simulink model "qbot2_sim_2019b"  (R2019b)
settings: Solver=FixedStepAuto  StartTime=0.0  StopTime=P.t_end  FixedStep=P.dt  RelTol=1e-3
InitFcn:
  | % load_qbot2_sim
StopFcn:
  | if (P.plotsim_flag)
  |     plot_sim(out, P)
  | end
(part 2 of 2)

== matlab function qbot2_sim_2019b/PVA Error State Estimation/Kalman Filter ==
  data: t_k input; f_b__i_b input; C_t__b input; v_t__t_b input; delta_r_t__t_b output; delta_v_t__t_b output; delta_C_t__b output; z_k_1 input; z_k_2 input; sigma_SNHT input; z_k_3 input; P parameter; P_posteriori_k output; residuals output; K output
function [delta_r_t__t_b, delta_v_t__t_b, delta_C_t__b, P_posteriori_k, residuals, K] = ...
              IMU_Error_State_Estimation(t_k, f_b__i_b, C_t__b, v_t__t_b, z_k_1, z_k_2, sigma_SNHT, z_k_3, P)

%% IMU Error State Estimation Function
% Recieves error measurements from the difference between odometry and the
% IMU, and provides estimates of that error.  

% Build randn quantities from etrinsic functions
coder.extrinsic('randn');

persistent x_posteriori_k_1 P_posteriori_k_1 A Q_bar K_prev

dt = P.dt;

% Normalize C_t__b_est
C_t__b = q2dcm(dcm2q(C_t__b));

%**************************************************************************
%% Kalman Filter Prediction Steps
%**************************************************************************

% For first instance only
if (isempty(x_posteriori_k_1))
    
    % Build Random Vector
    rand_vec = zeros(6,1);
    rand_vec = randn(6,1);
    
    % Set Initial Values for x and P_______________________________________
    P_0 = diag([5 * pi/180; 5 * pi/180; 5 * pi/180; ... % Initial Attitude Uncertianty (Angle-Axis)
                0.5; 0.5; 0.5; ...                      % Initial Velocity Uncertianty
                1.5; 1.5; 1.5; ...                      % Initial Position Uncertianty 
                10 * P.accel.BI.sigma_n; ...            % Initial Accel Bias Instability Uncertianty
                10 * P.gyro.BI.sigma_n] .^ 2);          % Initial Gyro Bias Instability Uncertianty
    x_0 = [z_k_2; ...                      % First measurement of attitude error
           z_k_1;   ...                    % First measurement of velocity error
           0; 0; 0;    ...                 % {t} frame always starts at zero
           ((P_0(10:15,10:15) / 10) * rand_vec)]; % Bias Instabilities drawn from distribution
    x_posteriori_k_1 = zeros(15,1);
    P_posteriori_k_1 = eye(15);
    
    K_prev = zeros(15,3);
    
    % Build the Contiuous Time Model_______________________________________
    A = zeros(15, 15);
    
    % Compute A - Fifth Row
    A(13:15, 13:15) = -eye(3) ./ P.gyro.BI.correlation_time;
    
    % Compute A - Fourth Row
    A(10:12, 10:12) = -eye(3) ./ P.accel.BI.correlation_time;
    
    % Compute A - Third Row
    A(7:9, 4:6) = eye(3);
    
    % Compute A - Second Row
    A(4:6, 1:3) = -vec2ss(C_t__b * f_b__i_b);
    A(4:6, 4:6) = -2 .* P.Ohm_t__i_e;
    A(4:6, 10:12) = -C_t__b;

    % Compute the monstrosity A(4:6, 7:9) a.k.a. A_23
    r_e__e_b_hat = P.r_e__e_t; % initial position is always the origin
    [L_b_hat, ~, ~] = xyz2llh(r_e__e_b_hat, P);
    g_0 = Somigliana(L_b_hat, P);
    r_e__e_S = Geo_Radius(L_b_hat, P);
    A(4:6, 7:9) = P.C_e__t' * ((2 * g_0 * r_e__e_b_hat) / ...
                 (r_e__e_S * norm(r_e__e_b_hat)^2)) * ...
                  r_e__e_b_hat' * P.C_e__t;
    
    % Compute A - First Row
    A(1:3, 1:3) = -P.Ohm_t__i_e;
    A(1:3, 13:15) = -C_t__b;
    
    % Define Q_bar_________________________________________________________
    Q_vec = [P.gyro.sigma_ARW.^2;   ...       % Attitude Process Noise rad/s
             P.accel.sigma_VRW.^2;  ...       % Velocity Process Noise m/s
             zeros(3,1);         ...          % Position Process Noise
             P.accel.BI.sigma_n.^2; ...       % Accel Bias Instability Process Noise m/s
             P.gyro.BI.sigma_n.^2];           % Gyro  Bias Instability Process Noise rad/s
     
    % Allow for a margin of error for tuning     
    Q_fudge_factor = 1;
    
    % Set Q
    Q_bar = diag(Q_fudge_factor .* Q_vec');
    
    % Discritize the Continuous Time Model_________________________________
    F = eye(15) + A*dt;
    Q = (1/2) * ((F*Q_bar*F') + Q_bar) * dt;
    
    % Compute first prediction_____________________________________________
    x_priori_k = F * x_0;
    P_priori_k = (F * P_0 * F') + Q;
    
%__________________________________________________________________________
% All other instances: State Prediction  
else
    
    % Re-compute the time varying arguements of A__________________________

    % Compute A - Second Row
    A(4:6, 1:3) = -vec2ss(C_t__b * f_b__i_b);
    A(4:6, 10:12) = -C_t__b;
    
    % Compute A - First Row
    A(1:3, 13:15) = -C_t__b;
    
    % Discritize the Continuous Time Model_________________________________
    F = eye(15) + A*dt;
    Q = (1/2) * ((F*Q_bar*F') + Q_bar) * dt;
    
    % Compute prediction step
    x_priori_k = (F * x_posteriori_k_1);
    P_priori_k = (F * P_posteriori_k_1 * F') + Q;
    
    % Symmetrisize P
    P_priori_k = (P_priori_k + P_priori_k') / 2;
    
end

%**************************************************************************
%% Kalman Filter Measurement Update Steps
%**************************************************************************
% This section is segmented according to the aiding sensor configuration

%__________________________________________________________________________
% No Measurement Updates
if (P.aiding_sensor_config == 0)
    
    x_posteriori_k = x_priori_k;
    P_posteriori_k = P_priori_k;
    residuals = zeros(3,1);
    K = zeros(15,3);
    
%__________________________________________________________________________
% Fake Velocity Aiding Only
elseif (P.aiding_sensor_config == 1)
    
    % Set H Matrix -- H = [(v_t__t_b,x), I_3, 0_3, 0_3, 0_3]
    H = [vec2ss(v_t__t_b), eye(3), zeros(3,9)]; 
    
    % Define R with known sigmas
    R_vec = P.sigma_fake_v .^ 2;
    R = diag(R_vec);
    
    % Kalman Gain Computation
    K = (P_priori_k * H') / (H * P_priori_k * H' + R);
    
    % Compute Residuals
    residuals = z_k_1 - H*x_priori_k;
    
    % A Posteriori State and Covariance Update
    x_posteriori_k = x_priori_k + K*(z_k_1 - H*x_priori_k);
    P_posteriori_k = (eye(15) - K*H) * P_priori_k;
    
    %Symmetrisize P
    P_posteriori_k = (P_posteriori_k + P_posteriori_k') / 2;
    

%__________________________________________________________________________
% Fake Attitude Only
elseif (P.aiding_sensor_config == 2)
    
    % Only Update at a frequency of 1 Hz
    if (mod(t_k, 1) == 0)
        
        % Set H Matrix -- H = [I_3, 0_3, 0_3, 0_3, 0_3]
        H = [eye(3), zeros(3,12)];
        
        % Define R with known sigmas
        R_vec = P.sigma_fake_psi .^ 2;
        R = diag(R_vec);
        
        % Kalman Gain Computation
        K = (P_priori_k * H') / (H * P_priori_k * H' + R);
        
        % Compute Residuals
        residuals = z_k_2 - H*x_priori_k;
        
        % A Posteriori State and Covariance Update
        x_posteriori_k = x_priori_k + K*(z_k_2 - H*x_priori_k);
        P_posteriori_k = (eye(15) - K*H) * P_priori_k;
        
        %Symmetrisize P
        P_posteriori_k = (P_posteriori_k + P_posteriori_k') / 2;
        
        % Save Value of K_prev
        K_prev = K;
    
    % No measurement update at this time step
    else
        
        % Carry Through
        x_posteriori_k = x_priori_k;
        P_posteriori_k = P_priori_k;
        residuals = zeros(3,1);
        K = K_prev;
       
    end
    

%__________________________________________________________________________
% Full Fake Attitude (Velocity & Attitude)
elseif (P.aiding_sensor_config == 3)
    
    % Velocity Update at every time step
    
    % Set H Matrix -- H = [(v_t__t_b,x), I_3, 0_3, 0_3, 0_3]
    H = [vec2ss(v_t__t_b), eye(3), zeros(3,9)];
    
    % Define R with known sigmas
    R_vec = P.sigma_fake_v .^ 2;
    R = diag(R_vec);
    
    % Kalman Gain Computation
    K = (P_priori_k * H') / (H * P_priori_k * H' + R);
    
    % Compute Residuals
    residuals = z_k_1 - H*x_priori_k;
    
    % A Posteriori State and Covariance Update
    x_posteriori_k = x_priori_k + K*(z_k_1 - H*x_priori_k);
    P_posteriori_k = (eye(15) - K*H) * P_priori_k;
    
    %Symmetrisize P
    P_posteriori_k = (P_posteriori_k + P_posteriori_k') / 2;
    
    %- - - - - - - - - - - - - - - - - - - - - - - - - - - - - - - - - - -
    % Attitude Update at a frequency of 1 Hz
    if (mod(t_k, 1) == 0)
        
        % Set H Matrix -- H = [I_3, 0_3, 0_3, 0_3, 0_3]
        H = [eye(3), zeros(3,12)];
        
        % Define R with known sigmas
        R_vec = P.sigma_fake_psi .^ 2;
        R = diag(R_vec);
        
        % Kalman Gain Computation
        K = (P_priori_k * H') / (H * P_priori_k * H' + R);
        
        % Compute Residuals
        residuals = z_k_2 - H*x_priori_k;
        
        % A Posteriori State and Covariance Update
        x_posteriori_k = x_priori_k + K*(z_k_2 - H*x_priori_k);
        P_posteriori_k = (eye(15) - K*H) * P_priori_k;
        
        %Symmetrisize P
        P_posteriori_k = (P_posteriori_k + P_posteriori_k') / 2;
        
        % Save Value of K_prev
        K_prev = K;
        
    end
    %- - - - - - - - - - - - - - - - - - - - - - - - - - - - - - - - - - -
    
%__________________________________________________________________________
% Odometry Aiding Only
elseif (P.aiding_sensor_config == 4)
    
    % Set H Matrix -- H = [(v_t__t_b,x), I_3, 0_3, 0_3, 0_3]
    H = [vec2ss(v_t__t_b), eye(3), zeros(3,9)]; 
    
    % Define R Vector
    R_b_vec = P.sigma_v_b__t_b_odo .^ 2;
    
    % Build the R Matrix
    R = C_t__b * diag(R_b_vec) * C_t__b';
    
    % Kalman Gain Computation
    K = (P_priori_k * H') / (H * P_priori_k * H' + R);
    
    % Compute Residuals
    residuals = z_k_1 - H*x_priori_k;
    
    % A Posteriori State and Covariance Update
    x_posteriori_k = x_priori_k + K*(z_k_1 - H*x_priori_k);
    P_posteriori_k = (eye(15) - K*H) * P_priori_k;
    
    %Symmetrisize P
    P_posteriori_k = (P_posteriori_k + P_posteriori_k') / 2;
    
%__________________________________________________________________________
% Kinect Camera Attitude Only
elseif (P.aiding_sensor_config == 5)
    
    % Only Update at a frequency of 1 Hz
    if (mod(t_k, 1) == 0)
        
        % Set H Matrix -- H = [I_3, 0_3, 0_3, 0_3, 0_3]
        H = [eye(3), zeros(3,12)];
        
        % Compute Jacobian
        [~, pitch, roll] = dcm2ypr(C_t__b);
        J = [1, 0, -sin(pitch); ...
             0, cos(roll), sin(roll)*cos(pitch); ...
             0, -sin(roll), cos(roll)*cos(pitch)];
        
        % Define R_e with known sigmas
        R_e = diag(sigma_SNHT .^ 2);
        
        % Convert R_e to R_k
        R_k = J * R_e * J';
        
        % Kalman Gain Computation
        K = (P_priori_k * H') / (H * P_priori_k * H' + R_k);
        
        % Compute Residuals
        residuals = z_k_2 - H*x_priori_k;
        
        % A Posteriori State and Covariance Update
        x_posteriori_k = x_priori_k + K*(z_k_2 - H*x_priori_k);
        P_posteriori_k = (eye(15) - K*H) * P_priori_k;
        
        %Symmetrisize P
        P_posteriori_k = (P_posteriori_k + P_posteriori_k') / 2;
        
        % Save Value of K_prev
        K_prev = K;
    
    % No measurement update at this time step
    else
        
        % Carry Through
        x_posteriori_k = x_priori_k;
        P_posteriori_k = P_priori_k;
        residuals = zeros(3,1);
        K = K_prev;
       
    end    

%__________________________________________________________________________
% Full Aiding (Odometry & Kinect Camera)
elseif (P.aiding_sensor_config == 6)
    
    % Velocity Update at every time step
    
    % Set H Matrix -- H = [(v_t__t_b,x), I_3, 0_3, 0_3, 0_3]
    H = [vec2ss(v_t__t_b), eye(3), zeros(3,9)];
    
    % Compute Jacobian
    [~, pitch, roll] = dcm2ypr(C_t__b);
    J = [1, 0, -sin(pitch); ...
         0, cos(roll), sin(roll)*cos(pitch); ...
         0, -sin(roll), cos(roll)*cos(pitch)];
    
    % Define R_e with known sigmas
    R_e = diag(sigma_SNHT .^ 2);
    
    % Convert R_e to R_k
    R_k = J * R_e * J';
    
    % Kalman Gain Computation
    K = (P_priori_k * H') / (H * P_priori_k * H' + R_k);
    
    % Compute Residuals
    residuals = z_k_1 - H*x_priori_k;
    
    % A Posteriori State and Covariance Update
    x_posteriori_k = x_priori_k + K*(z_k_1 - H*x_priori_k);
    P_posteriori_k = (eye(15) - K*H) * P_priori_k;
    
    %Symmetrisize P
    P_posteriori_k = (P_posteriori_k + P_posteriori_k') / 2;
    
    %- - - - - - - - - - - - - - - - - - - - - - - - - - - - - - - - - - -
    % Attitude Update at a frequency of 1 Hz
    if (mod(t_k, 1) == 0)
        
        % Set H Matrix -- H = [I_3, 0_3, 0_3, 0_3, 0_3]
        H = [eye(3), zeros(3,12)];
        
        % Define R with known sigmas
        R_vec = P.sigma_SNHT .^ 2;
        R = diag(R_vec);
        
        % Kalman Gain Computation
        K = (P_priori_k * H') / (H * P_priori_k * H' + R);
        
        % Compute Residuals
        residuals = z_k_2 - H*x_priori_k;
        
        % A Posteriori State and Covariance Update
        x_posteriori_k = x_priori_k + K*(z_k_2 - H*x_priori_k);
        P_posteriori_k = (eye(15) - K*H) * P_priori_k;
        
        %Symmetrisize P
        P_posteriori_k = (P_posteriori_k + P_posteriori_k') / 2;
        
        % Save Value of K_prev
        K_prev = K;
        
    end
    %- - - - - - - - - - - - - - - - - - - - - - - - - - - - - - - - - - -    
    
end

%__________________________________________________________________________
%% Barometer as an Aiding Sensor

if (P.use_barometer == true)
    
    % Set H (this is done as a one-dimensional case)
    H = 1;
    
    % Build the R Matrix
    R = P.sigma_baro^2 * 1.3;
    
    % Kalman Gain Computation
    P_priori_z = P_posteriori_k(9,9);
    K_baro = (P_priori_z * H') / (H * P_priori_z * H' + R);
    
    % A Posteriori State and Covariance Update
    x_posteriori_k(9) = x_priori_k(9) + K_baro*(z_k_3 - H*x_priori_k(9));
    P_posteriori_k(9,9) = (1 - K_baro*H) * P_priori_z;
    
    %Symmetrisize P
    P_posteriori_k = (P_posteriori_k + P_posteriori_k') / 2;
    
end
%__________________________________________________________________________
%% Pick-off State Estimates for Function Output

% State Estimates (AVP -> PVA)
delta_x_t__t_b_est = [x_posteriori_k(7:9); ...
                      x_posteriori_k(4:6); ...
                      x_posteriori_k(1:3)];

% Pull Off Position, Velocity, and Attitude Error Separately
delta_r_t__t_b = delta_x_t__t_b_est(1:3);
delta_v_t__t_b = delta_x_t__t_b_est(4:6);
delta_k_t__t_b = delta_x_t__t_b_est(7:9);

% Create and Normalize delta_C_t__b
delta_C_t__b = k2dcm(delta_k_t__t_b);
delta_C_t__b = q2dcm(dcm2q(delta_C_t__b));

%__________________________________________________________________________
%% Save State Estimates for Next Loop

x_posteriori_k_1 = x_posteriori_k;
P_posteriori_k_1 = P_posteriori_k;

end

== matlab function qbot2_sim_2019b/Odometry Stage 1/odo_pos_2_vel ==
  data: wheel_pos input; v_l output; v_r output; P parameter
%% Odometry True Position to Noisy Wheel Velocities
function [v_l, v_r]= pos2vel(wheel_pos, P)
                                                     
% Initialize Inital Conditions
persistent d_l_k_1 d_r_k_1

if (isempty(d_l_k_1))
    d_l_k_1 = 0;
    d_r_k_1 = 0;
end

% ISolate current wheel positions
d_l_k = wheel_pos(1,:);
d_r_k = wheel_pos(2,:);

% Build randn quantities from etrinsic functions
coder.extrinsic('randn');

% Preallocate Memory
randn1 = 0;
randn2 = 0;

% Build the randn variables
randn1 = randn;
randn2 = randn;

% Add Noise to Measurements if desired
if (P.odo_error_flag == true)
    d_l_k = d_l_k + P.sigma_odo_d * randn1;
    d_r_k = d_r_k + P.sigma_odo_d * randn2;
end

% Take this psuedo non-casual derivative
v_l = (d_l_k - d_l_k_1) / P.dt;
v_r = (d_r_k - d_r_k_1) / P.dt;

% Set the Current Values as the Previous Values
d_l_k_1 = d_l_k;
d_r_k_1 = d_r_k;

== matlab function qbot2_sim_2019b/Aiding Sensor Configurations/Fake Velocity Aiding Sensor ==
  data: Delta_v_t__t_b input; delta_fake_v_t__t_b_meas output; P parameter
function delta_fake_v_t__t_b_meas = fake_velocity_aiding_sensor(Delta_v_t__t_b, P)

% Set Up MATLAB's version of randn
coder.extrinsic('randn');

% Preallocate Memory
rand_vec = zeros(3,1);

% Call Randn Function
rand_vec = randn(3,1);

% Create Measurement Noise
noise_delta_v_t__t_b = P.sigma_fake_v .* rand_vec;

% Return Noisy Measurements
delta_fake_v_t__t_b_meas = Delta_v_t__t_b + noise_delta_v_t__t_b;

== matlab function qbot2_sim_2019b/Complimentary Filter/Angular Velocity Complimentary Filter ==
  data: w_b__i_b_meas input; w_t__t_b_imu output; w_t__t_b_odo input; w_t__t_b_odo output; w_t__t_b_comp output; w_t__t_b_lpf output; C_t__b_K output; P parameter
function [w_t__t_b_imu, w_t__t_b_odo, w_t__t_b_comp, w_t__t_b_lpf, C_t__b_K] = ...
          complimentary_filter(w_b__i_b_meas, w_t__t_b_odo, P)

% This block implments a complimentary filter between z-gyro measurements
% and odometry angular veocity measurements and then provides a corrected
% version of C_t__b_k

persistent C_t__b_K_1 delta_w_t__t_b_k_1 delta_w_t__t_b_lpf_k_1

% Initialize on First Time Step
if (isempty(C_t__b_K_1))
    
    % Use "truth" to initialize on first time step
    C_t__b_K  = eye(3);
    
    % Store current values as old values for next iteration
    C_t__b_K_1   = C_t__b_K;

    % Set Up Complimentary Filter Values
    delta_w_t__t_b_k_1 = zeros(3,1);
    delta_w_t__t_b_lpf_k_1 = zeros(3,1);
    
    % Return Other Output Values
    w_t__t_b_imu = C_t__b_K_1*w_b__i_b_meas - P.C_e__t'*P.w_i__i_e;
    w_t__t_b_comp = w_t__t_b_imu;
    w_t__t_b_lpf = w_t__t_b_imu;
    
%% For all other time steps
else
    
    % Employ Complimentary Filter__________________________________________
    if (P.use_comp_filter == true)
        
        % Calculate w_t__t_b_imu
        w_t__t_b_imu = C_t__b_K_1*w_b__i_b_meas - P.C_e__t'*P.w_i__i_e;
        
        % Take the difference between the odo and imu measurements
        delta_w_t__t_b = w_t__t_b_odo - w_t__t_b_imu;
        
        % Pass the w error through the Low Pass Filter (LPF)
        w_t__t_b_lpf = -P.lpf_den_1 .* delta_w_t__t_b_lpf_k_1 + ...
                        P.lpf_num_1 .* delta_w_t__t_b + ...
                        P.lpf_num_2 .* delta_w_t__t_b_k_1;
        
        % Sum up the LPF'd error and IMU meas
        w_t__t_b_comp = w_t__t_b_imu + w_t__t_b_lpf;
        
        % Catch for when w_t__t_b is super super small
        if (norm(w_t__t_b_comp) < (5 * eps))
            C_t__b_K = C_t__b_K_1;
        else
            C_t__b_K = Rodrigues_k(w_t__t_b_comp * P.dt) * C_t__b_K_1;
        end
    
    % If not using Complimentary Filter____________________________________
    else
   
        % Calculate w_t__t_b_imu
        w_t__t_b_imu = C_t__b_K_1*w_b__i_b_meas - P.C_e__t'*P.w_i__i_e;
        
        % Catch for when w_t__t_b is super super small
        if (norm(w_t__t_b_imu) < (5 * eps))
            C_t__b_K = C_t__b_K_1;
        else
            C_t__b_K = Rodrigues_k(w_t__t_b_imu * P.dt) * C_t__b_K_1;
        end
        
        % Return zeros for comp filter variables
        w_t__t_b_comp = zeros(3,1);
        w_t__t_b_lpf = zeros(3,1);
        delta_w_t__t_b = zeros(3,1);
        delta_w_t__t_b_k_1 = zeros(3,1);
        delta_w_t__t_b_lpf_k_1 = zeros(3,1);
        
    end
    
    % Normalize C_t__b_K___________________________________________________
    C_t__b_K = q2dcm(dcm2q(C_t__b_K));
    
    
% Store New Value as the Old_______________________________________________
C_t__b_K_1 = C_t__b_K;
delta_w_t__t_b_k_1 = delta_w_t__t_b;
delta_w_t__t_b_lpf_k_1 = w_t__t_b_lpf;

end

== matlab function qbot2_sim_2019b/Aiding Sensor Configurations/Odometry Stage 2/Rotate_Speed ==
  data: C_t__b_k input; v_t__t_b_odo output; v_b__t_b_odo input
function v_t__t_b_odo = rotate_speed(C_t__b_k, v_b__t_b_odo)

% Rotate Speed in the body frame into the {t} frame
v_t__t_b_odo = C_t__b_k * v_b__t_b_odo;

== matlab function qbot2_sim_2019b/Aiding Sensor Configurations/Fake Attitude Aiding Sensor ==
  data: Delta_euler_t__t_b input; delta_fake_psi_t__t_b_meas output; P parameter
function delta_fake_psi_t__t_b_meas = fake_aiding_sensor(Delta_euler_t__t_b, P)

% Set Up MATLAB's version of randn
coder.extrinsic('randn');

% Preallocate Memory
rand_vec = zeros(3,1);

% Call Randn Function
rand_vec = randn(3,1);

% Create Measurement Noise
noise_delta_psi_t__t_b = P.sigma_fake_psi .* rand_vec;

% Convert Euler Truth to Angle-Axis
Delta_psi_t__t_b = dcm2k(ypr2dcm(Delta_euler_t__t_b(3), ...
                                 Delta_euler_t__t_b(2), ...
                                 Delta_euler_t__t_b(1)));

% Create Noisy Euler Angle Measurements
delta_fake_psi_t__t_b_meas = Delta_psi_t__t_b + noise_delta_psi_t__t_b;

== matlab function qbot2_sim_2019b/Barometer Measurement Simulation/Barometer Simulator ==
  data: height_true input; height_meas output; P parameter
function height_meas = baro_sim(height_true, P)

% Build randn quantities from etrinsic functions
coder.extrinsic('randn');

% Compute Barometer Error
baro_error = 0;
baro_error = P.sigma_baro * randn;

% Add Error to True Height
height_meas = height_true + baro_error;

== matlab function qbot2_sim_2019b/Aiding Sensor Configurations/Kalman Filter Measurement Seletion ==
  data: delta_fake_v_t__t_b_meas input; z_k_1 output; delta_fake_psi_t__t_b_meas input; delta_v_t__t_b_meas input; delta_k_t__t_b_meas input; P parameter; z_k_2 output
function [z_k_1, z_k_2]  = KF_meas_select(delta_fake_v_t__t_b_meas, ...
                                          delta_fake_psi_t__t_b_meas, ...
                                          delta_v_t__t_b_meas, ...
                                          delta_k_t__t_b_meas, ...
                                          P)
                                      
% Selects measurements for the Kalman Filter

% No Measurement Update
if (P.aiding_sensor_config == 0)
    z_k_1 = zeros(3,1);
    z_k_2 = zeros(3,1);

% Fake Velocity Aiding Only
elseif (P.aiding_sensor_config == 1)
    z_k_1 = delta_fake_v_t__t_b_meas;
    z_k_2 = zeros(3,1);
    
% Fake Attitude Aiding Only    
elseif (P.aiding_sensor_config == 2)
    z_k_1 = zeros(3,1); 
    z_k_2 = delta_fake_psi_t__t_b_meas;

% Full Fake Aiding (Attitude & Velocity)    
elseif (P.aiding_sensor_config == 3)
    z_k_1 = delta_fake_v_t__t_b_meas;
    z_k_2 = delta_fake_psi_t__t_b_meas;    
    
% Odometry Only    
elseif (P.aiding_sensor_config == 4)
    z_k_1 = delta_v_t__t_b_meas;
    z_k_2 = zeros(3,1);

% Kinect Camera Aiding Only
elseif (P.aiding_sensor_config == 5)
    z_k_1 = zeros(3,1);
    z_k_2 = delta_k_t__t_b_meas;
    
% Full Aiding (Odometry & Kinect Camera) Aiding Only
elseif (P.aiding_sensor_config == 6)
    z_k_1 = delta_v_t__t_b_meas;
    z_k_2 = delta_k_t__t_b_meas;    
    
else
    error("No Valid Aiding Sensor Configuration Selected")
    
end

end

== matlab function qbot2_sim_2019b/Kinect Camera Attitude Memeasurement Simulation/Kinect Camera Sim ==
  data: t input; psi_t__t_b input; C_t__b_kinect output; P parameter; sigma_SNHT output
function [C_t__b_kinect, sigma_SNHT] = kinect_camera_sim(t, psi_t__t_b, P)

% Build randn quantities from etrinsic functions
coder.extrinsic('randn');

% Preallocate Memory
randn1 = 0;
randn2 = 0;

% Set Random Values via the randn external function
randn1 = randn;
randn2 = randn;

if (mod(t, 1) == 0)
    
    % Take Ground Truth Measurements and Create Simulated C_t__b_Measurements
    theta_true = 0;
    psi_true = psi_t__t_b(3);
    
    % Add Noise to Ground Truth
    theta_meas = theta_true + (P.sigma_pitch * randn1);
    psi_meas = psi_true + (P.sigma_yaw * randn2);
    
    % Convert Noisy Euler Angles into a DCM
    C_t__b_kinect = ypr2dcm(psi_meas, theta_meas, 0);
    
    % Change Up the sigma_SNHT each time-step a little bit
    sigma_SNHT = P.sigma_SNHT;
%     sigma_SNHT = [P.sigma_SNHT(1) + (2.5*randn4); ...
%                   P.sigma_SNHT(2) + (2.5*randn5); ...
%                   P.sigma_SNHT(3) + (2.5*randn6)];
        
else
    
    C_t__b_kinect = eye(3);
    sigma_SNHT = zeros(3,1);
    
end

== matlab function qbot2_sim_2019b/Aiding Sensor Configurations/kinect_attitude_reconclie ==
  data: C_t__b_comp input; delta_k_t__t_b_meas output; C_t__b_kinect input; t input
function delta_k_t__t_b_meas = kinect_attitude_reconcile(C_t__b_comp, C_t__b_kinect, t)

if (mod(t, 1) == 0)
    
    % Find the error via dC = C1 * C2^T
    delta_C_t__b_meas = C_t__b_kinect * C_t__b_comp';
    
    % Convert Error in DCM to Error in Angle-Axis
    delta_k_t__t_b_meas = dcm2k(delta_C_t__b_meas);
    
else
    
    delta_k_t__t_b_meas = [0; 0; 0];
    
end
